simulink model "Repetitive_Controller_2"  (R2021b)
settings: Solver=VariableStepAuto  StartTime=0.0  StopTime=tspan(2)  RelTol=1e-9
undefined symbols (not defined in the file): K1, K2, RC_gain_x, RC_gain_y, T_x, T_y, Tau_T_beta, Tau_T_gamma, Tau_x, Tau_y, Tmax
libraries: cstblocks x2
settings Model: Creator=domin  LastModifiedBy=domin
settings DebuggingCC: ModelReferenceExtraNoncontSigs=none

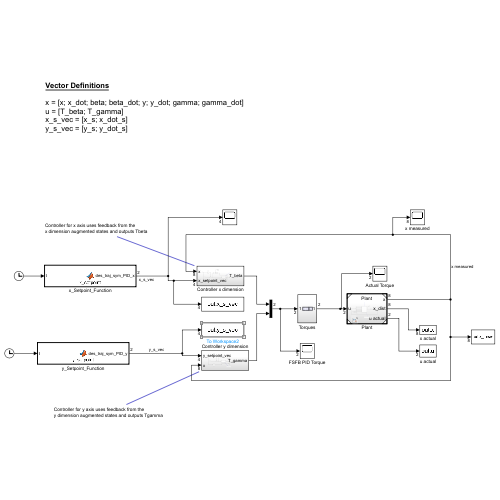
[thumbnail: Simulink's stored preview of the top-level diagram]
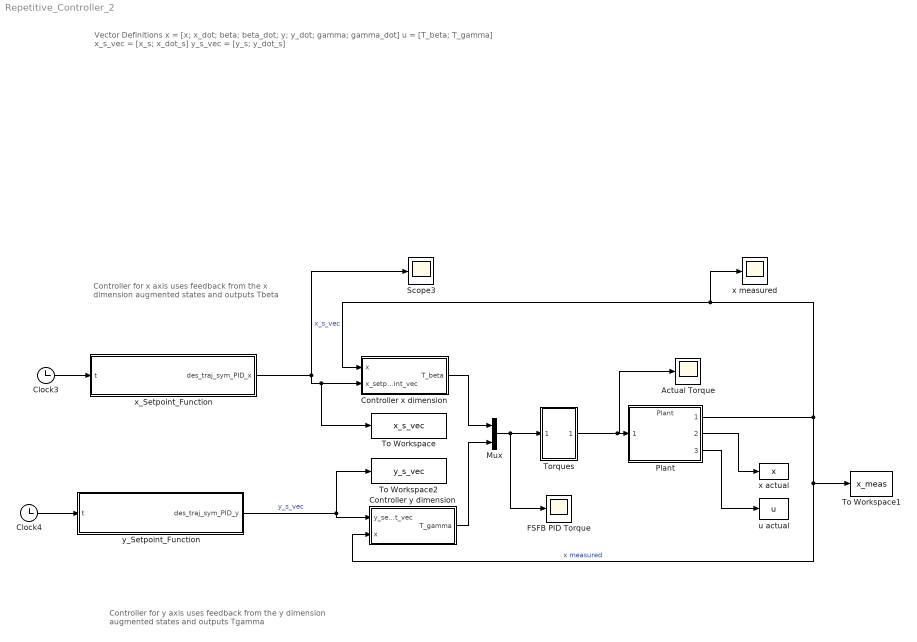
== system Repetitive_Controller_2 ==
  note: Controller for y axis uses feedback from the
      | y dimension augmented states and outputs Tgamma
  note: Controller for x axis uses feedback from the
      | x dimension augmented states and outputs Tbeta
  note: Vector Definitions
      |
      | x = [x; x_dot; beta; beta_dot; y; y_dot; gamma; gamma_dot]
      | u = [T_beta; T_gamma]
      | x_s_vec = [x_s; x_dot_s]
      | y_s_vec = [y_s; y_dot_s]
  Actual Torque : Scope
  Clock3 : Clock
  Clock4 : Clock
  Controller x dimension : Subsystem
  Controller y dimension : Subsystem
  FSFB PID Torque : Scope
  Mux : Mux  Inputs=2
  Plant : ModelReference  ModelNameDialog=Plant  SimulationMode=Normal  ModelReferenceVersion=1.53
  Scope3 : Scope
  To Workspace : ToWorkspace  VariableName=x_s_vec  SampleTime=-1
  To Workspace1 : ToWorkspace  VariableName=x_meas  SampleTime=-1
  To Workspace2 : ToWorkspace  VariableName=y_s_vec  SampleTime=-1
  Torques : Subsystem
  u actual : ToWorkspace  VariableName=u  SampleTime=-1
  x actual : ToWorkspace  VariableName=x  SampleTime=-1
  x measured : Scope
  x_Setpoint_Function : MATLAB Function  TreatAsAtomicUnit=on
  y_Setpoint_Function : MATLAB Function  TreatAsAtomicUnit=on
  wires:
  Controller x dimension/1(T_beta) -> Mux/1
  Mux/1 -> Torques/1(In1), FSFB PID Torque/1
  Controller y dimension/1(T_gamma) -> Mux/2
  Torques/1(Out2) -> Actual Torque/1, Plant/1
  Plant/3 -> u actual/1
  Plant/2 -> x actual/1
  Plant/1 -> Controller x dimension/1(x), x measured/1, Controller y dimension/2(x), To Workspace1/1  "x measured"
  Clock4/1 -> y_Setpoint_Function/1(t)
  y_Setpoint_Function/1(des_traj_sym_PID_y) -> Controller y dimension/1(y_setpoint_vec), To Workspace2/1  "y_s_vec"
  x_Setpoint_Function/1(des_traj_sym_PID_x) -> Controller x dimension/2(x_setpoint_vec), To Workspace/1, Scope3/1  "x_s_vec"
  Clock3/1 -> x_Setpoint_Function/1(t)

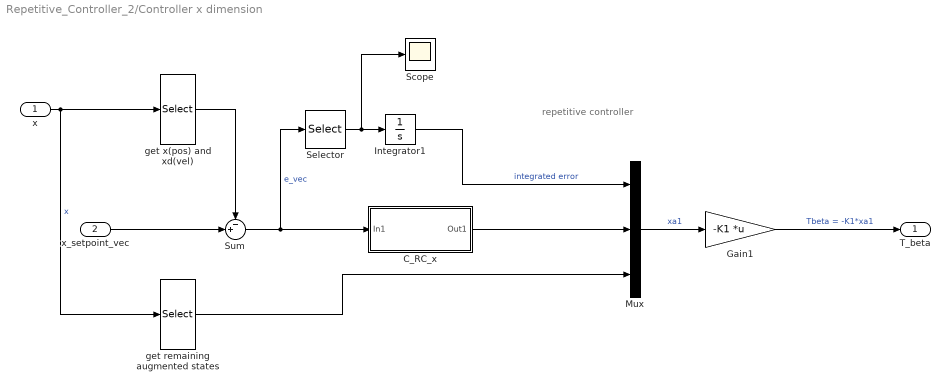
== system Repetitive_Controller_2/Controller x dimension ==
  note: repetitive controller
  x : Inport
  x_setpoint_vec : Inport  Port=2
  C_RC_x : Subsystem
  Gain1 : Gain  Gain=-K1  Multiplication=Matrix(K*u)
  Integrator1 : Integrator
  Mux : Mux  Inputs=3
  Scope : Scope
  Selector : Selector  InputPortWidth=2  IndexOptions=Index vector (dialog)  Indices=[1 ]  OutputSizes=1
  Sum : Sum  Inputs=-+|
  get remaining augmented states : Selector  InputPortWidth=8  IndexOptions=Index vector (dialog)  Indices=[3,4]  OutputSizes=1
  get x(pos) and xd(vel) : Selector  InputPortWidth=8  IndexOptions=Index vector (dialog)  Indices=[1 2]  OutputSizes=1
  T_beta : Outport
  wires:
  get remaining augmented states/1 -> Mux/3
  Gain1/1 -> T_beta/1  "Tbeta = -K1*xa1"
  get x(pos) and xd(vel)/1 -> Sum/1
  Mux/1 -> Gain1/1  "xa1"
  Sum/1 -> Selector/1, C_RC_x/1(In1)  "e_vec"
  x_setpoint_vec/1 -> Sum/2
  x/1 -> get x(pos) and xd(vel)/1, get remaining augmented states/1  "x"
  Selector/1 -> Scope/1, Integrator1/1
  Integrator1/1 -> Mux/1  "integrated error"
  C_RC_x/1(Out1) -> Mux/2

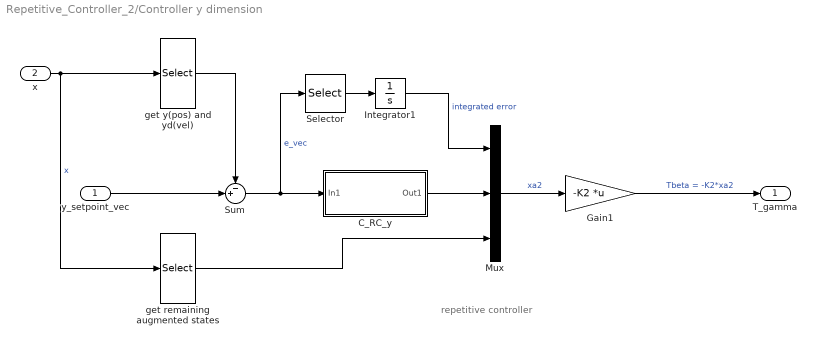
== system Repetitive_Controller_2/Controller y dimension ==
  note: repetitive controller
  y_setpoint_vec : Inport
  x : Inport  Port=2
  C_RC_y : Subsystem
  Gain1 : Gain  Gain=-K2  Multiplication=Matrix(K*u)
  Integrator1 : Integrator
  Mux : Mux  Inputs=3
  Selector : Selector  InputPortWidth=2  IndexOptions=Index vector (dialog)  Indices=[1 ]  OutputSizes=1
  Sum : Sum  Inputs=-+|
  get remaining augmented states : Selector  InputPortWidth=8  IndexOptions=Index vector (dialog)  Indices=[7,8]  OutputSizes=1
  get y(pos) and yd(vel) : Selector  InputPortWidth=8  IndexOptions=Index vector (dialog)  Indices=[5 6]  OutputSizes=1
  T_gamma : Outport
  wires:
  Integrator1/1 -> Mux/1  "integrated error"
  x/1 -> get y(pos) and yd(vel)/1, get remaining augmented states/1  "x"
  Gain1/1 -> T_gamma/1  "Tbeta = -K2*xa2"
  get y(pos) and yd(vel)/1 -> Sum/1
  Mux/1 -> Gain1/1  "xa2"
  get remaining augmented states/1 -> Mux/3
  Selector/1 -> Integrator1/1
  Sum/1 -> Selector/1, C_RC_y/1(In1)  "e_vec"
  y_setpoint_vec/1 -> Sum/2
  C_RC_y/1(Out1) -> Mux/2

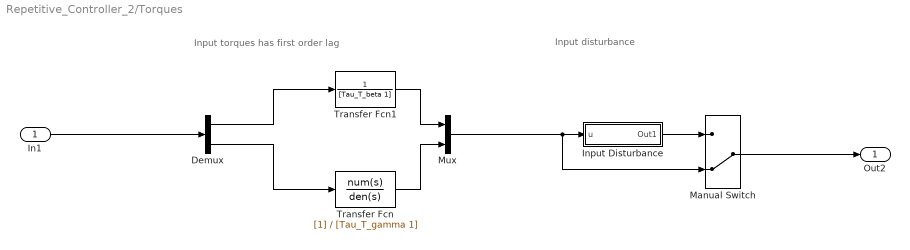
== system Repetitive_Controller_2/Torques ==
  note: Input disturbance
  note: Input torques has first order lag
  In1 : Inport
  Demux : Demux  Outputs=2
  Input Disturbance : Subsystem
  Manual Switch : ManualSwitch  CurrentSetting=0
  Mux : Mux  Inputs=2
  Transfer Fcn : TransferFcn  Denominator=[Tau_T_gamma 1]
  Transfer Fcn1 : TransferFcn  Denominator=[Tau_T_beta 1]
  Out2 : Outport
  wires:
  In1/1 -> Demux/1
  Demux/1 -> Transfer Fcn1/1
  Transfer Fcn/1 -> Mux/2
  Demux/2 -> Transfer Fcn/1
  Transfer Fcn1/1 -> Mux/1
  Input Disturbance/1(Out1) -> Manual Switch/1
  Mux/1 -> Manual Switch/2, Input Disturbance/1(u)
  Manual Switch/1 -> Out2/1

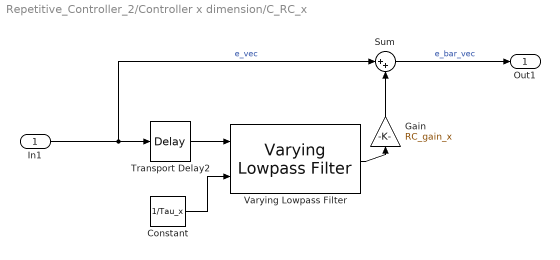
== system Repetitive_Controller_2/Controller x dimension/C_RC_x ==
  In1 : Inport
  Constant : Constant  Value=1/Tau_x
  Gain : Gain  Gain=RC_gain_x
  Sum : Sum  Inputs=|++
  Transport Delay2 : TransportDelay  DelayTime=T_x  BufferSize=100000
  Varying Lowpass Filter : cstblocks/Linear Parameter Varying/Varying Lowpass Filter  N=1
  Out1 : Outport
  wires:
  In1/1 -> Sum/1, Transport Delay2/1  "e_vec"
  Transport Delay2/1 -> Varying Lowpass Filter/1
  Varying Lowpass Filter/1 -> Gain/1
  Sum/1 -> Out1/1  "e_bar_vec"
  Constant/1 -> Varying Lowpass Filter/2
  Gain/1 -> Sum/2

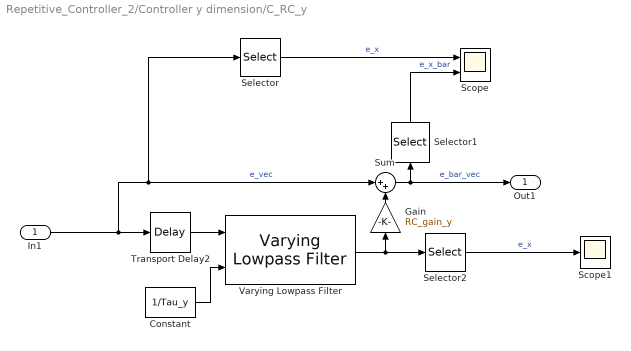
== system Repetitive_Controller_2/Controller y dimension/C_RC_y ==
  In1 : Inport
  Constant : Constant  Value=1/Tau_y
  Gain : Gain  Gain=RC_gain_y
  Scope : Scope  NumInputPorts=2
  Scope1 : Scope
  Selector : Selector  InputPortWidth=2  IndexOptions=Index vector (dialog)  Indices=[1]  OutputSizes=1
  Selector1 : Selector  InputPortWidth=2  IndexOptions=Index vector (dialog)  Indices=[1]  OutputSizes=1
  Selector2 : Selector  InputPortWidth=2  IndexOptions=Index vector (dialog)  Indices=[1]  OutputSizes=1
  Sum : Sum  Inputs=|++
  Transport Delay2 : TransportDelay  DelayTime=T_y  BufferSize=100000
  Varying Lowpass Filter : cstblocks/Linear Parameter Varying/Varying Lowpass Filter  N=1
  Out1 : Outport
  wires:
  In1/1 -> Selector/1, Sum/1, Transport Delay2/1  "e_vec"
  Transport Delay2/1 -> Varying Lowpass Filter/1
  Varying Lowpass Filter/1 -> Gain/1, Selector2/1
  Sum/1 -> Selector1/1, Out1/1  "e_bar_vec"
  Constant/1 -> Varying Lowpass Filter/2
  Selector/1 -> Scope/1  "e_x"
  Selector1/1 -> Scope/2  "e_x_bar"
  Gain/1 -> Sum/2
  Selector2/1 -> Scope1/1  "e_x"

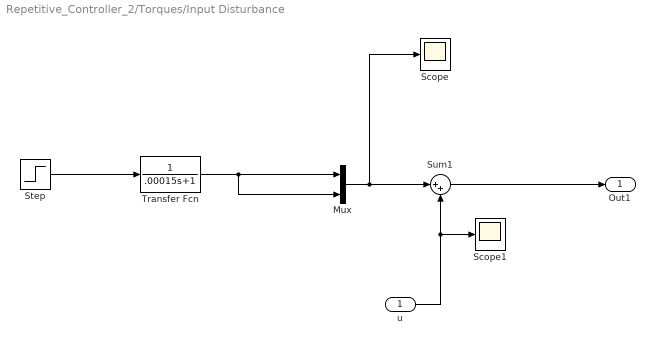
== system Repetitive_Controller_2/Torques/Input Disturbance ==
  u : Inport
  Mux : Mux  Inputs=2
  Scope : Scope
  Scope1 : Scope
  Step : Step  Time=10  After=Tmax/2  SampleTime=0
  Sum1 : Sum  Inputs=|++
  Transfer Fcn : TransferFcn  Denominator=[.00015 1]
  Out1 : Outport
  wires:
  Step/1 -> Transfer Fcn/1
  Sum1/1 -> Out1/1
  Transfer Fcn/1 -> Mux/2, Mux/1
  Mux/1 -> Scope/1, Sum1/1
  u/1 -> Scope1/1, Sum1/2

== matlab function Repetitive_Controller_2/y_Setpoint_Function ==
  data: t input; des_traj_sym_PID_y output
function des_traj_sym_PID_y = y_setpoint(t)
%#codegen

%    This function was generated by the Symbolic Math Toolbox version 9.0.
%    06-Feb-2022 18:29:46

t2 = pi./2.0;
t3 = t./2.0;
t4 = t.*pi.*(2.0./3.0);
t5 = -t3;
t8 = t2+t4;
t6 = exp(t5);
t9 = sin(t8);
t7 = t6-1.0;
des_traj_sym_PID_y = [t7.*t9.*(-1.0./5.0);(t6.*t9)./1.0e+1-t7.*pi.*cos(t8).*(2.0./1.5e+1)];

== matlab function Repetitive_Controller_2/x_Setpoint_Function ==
  data: t input; des_traj_sym_PID_x output
function des_traj_sym_PID_x = x_setpoint(t)
%#codegen

%    This function was generated by the Symbolic Math Toolbox version 9.0.
%    06-Feb-2022 18:29:46

t2 = t./2.0;
t3 = t.*pi.*(2.0./3.0);
t4 = -t2;
t6 = sin(t3);
t5 = exp(t4);
t7 = t5-1.0;
des_traj_sym_PID_x = [t6.*t7.*(-1.0./5.0);(t5.*t6)./1.0e+1-t7.*pi.*cos(t3).*(2.0./1.5e+1)];
